simulink model "CryoDet6"  (R2015a)
settings: Solver=ode45  SolverMode=SingleTasking  StartTime=0.0  StopTime=1e-3  MaxStep=Tclk/8  RelTol=1e-3
values from neighbouring files (symbols this model uses):
  Fclk = Fadc/2    (= 185000000)    [setupCryoFPGA.m]    (also in setupCryoNew.m)
  noise = exp(1i*phi)    [setupCryoFPGA.m]    (also in setupCryoNew.m = exp(2i*pi*rand(1, noiseLen)))
  noiseLen = 128    [setupCryoFPGA.m]    (also in setupCryoNew.m)
  noiseSteps = 32    [setupCryoFPGA.m]    (also in setupCryoNew.m)
  notch = tf( [1 a*wNotch/Q wNotch^2], [1 wNotch/Q wNotch^2])    [setupCryoFPGA.m]    (also in setupCryoNew.m)
  notch2 = tf( [1 a*wNotch/Q wNotch^2], [1 wNotch/Q wNotch^2])    [setupCryoFPGA.m]    (also in setupCryoNew.m)
  setupVers = 5    [setupCryoFPGA.m]    (also in setupCryoNew.m = 21)
  Tclk = 1/Fclk    (= 5.40540540541e-09)    [setupCryoFPGA.m]    (also in setupCryoNew.m)
  wTs1 = w1*Ts1    (= 0.0271705310581)    [setupCryoFPGA.m]
undefined symbols (not defined in the file or in its folder): AXI4, Lite, xlipgetpartsetting
libraries: xbsIndex_r4 x516, simulink x1
(part 4 of 6)

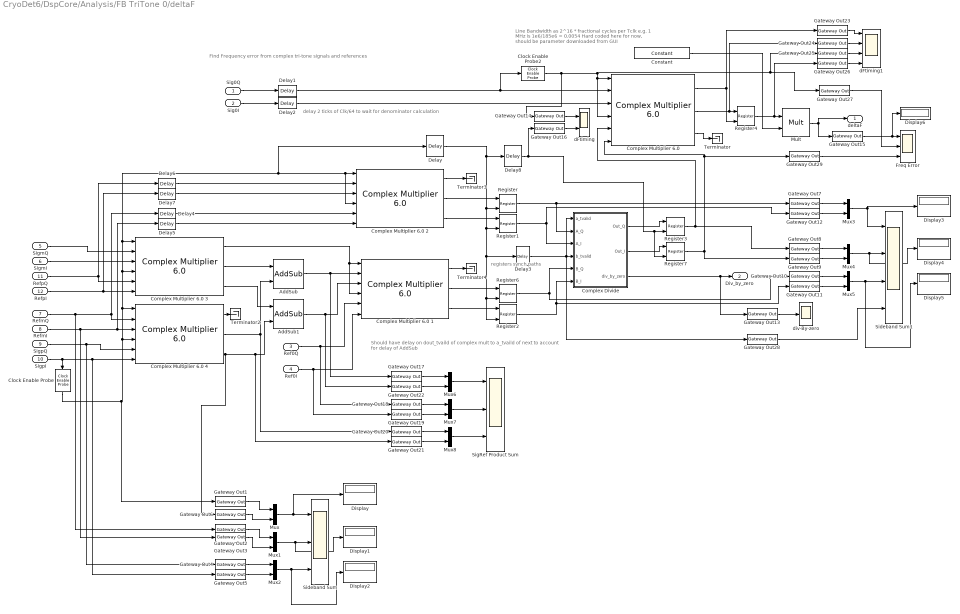
== system CryoDet6/DspCore/Analysis/FB TriTone 0/deltaF ==
  note: Should have delay on dout_tvaild of complex mult to a_tvaild of next
      | to account for delay of AddSub
  note: registers
      | synch
      | paths
  note: delay 2 ticks of Clk/64 to wait for denominator calculation
  note: Line Bandwidth as 2^16 * fractional cycles per Tclk
      | e.g. 1 MHz is 1e6/185e6 = 0.0054
      | Hard coded here for now, should be parameter
      | downloaded from GUI
  note: Find Frequency error from complex tri-tone signals and references
  Sig0Q : Inport
  Sig0I : Inport  Port=2
  Ref0Q : Inport  Port=3
  Ref0I : Inport  Port=4
  SigmQ : Inport  Port=5
  SigmI : Inport  Port=6
  RefmQ : Inport  Port=7
  RefmI : Inport  Port=8
  SigpQ : Inport  Port=9
  SigpI : Inport  Port=10
  RefpQ : Inport  Port=11
  RefpI : Inport  Port=12
  AddSub : xbsIndex_r4/AddSub  mode=Addition  use_carryin=off  use_carryout=off  en=off  latency=3  precision=User Defined  arith_type="Signed  (2's comp)"  n_bits=32  bin_pt=30  quantization=Truncate  overflow=Wrap  use_behavioral_HDL=off  hw_selection=Fabric  pipelined=off  dbl_ovrd=off  block_type=addsub
  AddSub1 : xbsIndex_r4/AddSub  mode=Addition  use_carryin=off  use_carryout=off  en=off  latency=3  precision=User Defined  arith_type="Signed  (2's comp)"  n_bits=32  bin_pt=30  quantization=Truncate  overflow=Wrap  use_behavioral_HDL=off  hw_selection=Fabric  pipelined=off  dbl_ovrd=off  block_type=addsub
  Clock Enable Probe : xbsIndex_r4/Clock Enable Probe  inherit_constraints=on  block_type=ceprobe
      settings: infoedit="Clock enable extractor.  Produces a Boolean output that mirrors the hardware clock enable associated with the input sample rate.<br><br>Hardware notes: in hardware this block costs nothing."
  Clock Enable Probe2 : xbsIndex_r4/Clock Enable Probe  inherit_constraints=on  block_type=ceprobe
      settings: infoedit="Clock enable extractor.  Produces a Boolean output that mirrors the hardware clock enable associated with the input sample rate.<br><br>Hardware notes: in hardware this block costs nothing."
  Complex Divide : Subsystem
  "Complex Multiplier 6.0 " : xbsIndex_r4/Complex Multiplier 6.0   hasatlast=off  hasatuser=off  atuserwidth=1  hasbtlast=off  hasbtuser=off  btuserwidth=1  multtype=Use_Mults  optimizegoal=Resources  flowcontrol=NonBlocking  outputwidth=33  roundmode=Truncate  hasctrltlast=off  hasctrltuser=off  ctrltuserwidth=1  outtlastbehv=Null  latencyconfig=Manual  minimumlatency=37  aclken=off  aresetn=off  trim_axipin_name=on  simulation_type=hybrid_sim  simulation_model=sysgen:cmpy_v6_0  data_path_portlist={ 's_axis_a_tdata_real', 's_axis_a_tdata_imag', 's_axis_b_tdata_real', 's_axis_b_tdata_imag', 's_axis_ctrl_tdata_rounding_bit', 'm_axis_dout_tdata_real', 'm_axis_dout_tdata_imag' }  aportwidth=63  bportwidth=63  ip_name=Complex Multiplier  ip_version=6.0  dsptool_ready=true  ipcore_usecache=true  ipcore_useipmodelcache=true  ipcore_verbose=false  ipcore_latency_parameter='minimumlatency'  wrapper_available=true  port_translation_map={ 'aclken' => 'en', 'aresetn' => 'rst'}  block_type=cmpy_v6_0
  Complex Multiplier 6.0 1 : xbsIndex_r4/Complex Multiplier 6.0   hasatlast=off  hasatuser=off  atuserwidth=1  hasbtlast=off  hasbtuser=off  btuserwidth=1  multtype=Use_Mults  optimizegoal=Resources  flowcontrol=NonBlocking  outputwidth=48  roundmode=Truncate  hasctrltlast=off  hasctrltuser=off  ctrltuserwidth=1  outtlastbehv=Null  latencyconfig=Manual  minimumlatency=37  aclken=off  aresetn=off  trim_axipin_name=on  simulation_type=hybrid_sim  simulation_model=sysgen:cmpy_v6_0  data_path_portlist={ 's_axis_a_tdata_real', 's_axis_a_tdata_imag', 's_axis_b_tdata_real', 's_axis_b_tdata_imag', 's_axis_ctrl_tdata_rounding_bit', 'm_axis_dout_tdata_real', 'm_axis_dout_tdata_imag' }  aportwidth=63  bportwidth=63  ip_name=Complex Multiplier  ip_version=6.0  dsptool_ready=true  ipcore_usecache=true  ipcore_useipmodelcache=true  ipcore_verbose=false  ipcore_latency_parameter='minimumlatency'  wrapper_available=true  port_translation_map={ 'aclken' => 'en', 'aresetn' => 'rst'}  block_type=cmpy_v6_0
  Complex Multiplier 6.0 2 : xbsIndex_r4/Complex Multiplier 6.0   hasatlast=off  hasatuser=off  atuserwidth=1  hasbtlast=off  hasbtuser=off  btuserwidth=1  multtype=Use_Mults  optimizegoal=Resources  flowcontrol=NonBlocking  outputwidth=32  roundmode=Truncate  hasctrltlast=off  hasctrltuser=off  ctrltuserwidth=1  outtlastbehv=Null  latencyconfig=Manual  minimumlatency=37  aclken=off  aresetn=off  trim_axipin_name=on  simulation_type=hybrid_sim  simulation_model=sysgen:cmpy_v6_0  data_path_portlist={ 's_axis_a_tdata_real', 's_axis_a_tdata_imag', 's_axis_b_tdata_real', 's_axis_b_tdata_imag', 's_axis_ctrl_tdata_rounding_bit', 'm_axis_dout_tdata_real', 'm_axis_dout_tdata_imag' }  aportwidth=63  bportwidth=63  ip_name=Complex Multiplier  ip_version=6.0  dsptool_ready=true  ipcore_usecache=true  ipcore_useipmodelcache=true  ipcore_verbose=false  ipcore_latency_parameter='minimumlatency'  wrapper_available=true  port_translation_map={ 'aclken' => 'en', 'aresetn' => 'rst'}  block_type=cmpy_v6_0
  Complex Multiplier 6.0 3 : xbsIndex_r4/Complex Multiplier 6.0   hasatlast=off  hasatuser=off  atuserwidth=1  hasbtlast=off  hasbtuser=off  btuserwidth=1  multtype=Use_Mults  optimizegoal=Resources  flowcontrol=NonBlocking  outputwidth=32  roundmode=Truncate  hasctrltlast=off  hasctrltuser=off  ctrltuserwidth=1  outtlastbehv=Null  latencyconfig=Manual  minimumlatency=37  aclken=off  aresetn=off  trim_axipin_name=on  simulation_type=hybrid_sim  simulation_model=sysgen:cmpy_v6_0  data_path_portlist={ 's_axis_a_tdata_real', 's_axis_a_tdata_imag', 's_axis_b_tdata_real', 's_axis_b_tdata_imag', 's_axis_ctrl_tdata_rounding_bit', 'm_axis_dout_tdata_real', 'm_axis_dout_tdata_imag' }  aportwidth=63  bportwidth=63  ip_name=Complex Multiplier  ip_version=6.0  dsptool_ready=true  ipcore_usecache=true  ipcore_useipmodelcache=true  ipcore_verbose=false  ipcore_latency_parameter='minimumlatency'  wrapper_available=true  port_translation_map={ 'aclken' => 'en', 'aresetn' => 'rst'}  block_type=cmpy_v6_0
  Complex Multiplier 6.0 4 : xbsIndex_r4/Complex Multiplier 6.0   hasatlast=off  hasatuser=off  atuserwidth=1  hasbtlast=off  hasbtuser=off  btuserwidth=1  multtype=Use_Mults  optimizegoal=Resources  flowcontrol=NonBlocking  outputwidth=32  roundmode=Truncate  hasctrltlast=off  hasctrltuser=off  ctrltuserwidth=1  outtlastbehv=Null  latencyconfig=Manual  minimumlatency=37  aclken=off  aresetn=off  trim_axipin_name=on  simulation_type=hybrid_sim  simulation_model=sysgen:cmpy_v6_0  data_path_portlist={ 's_axis_a_tdata_real', 's_axis_a_tdata_imag', 's_axis_b_tdata_real', 's_axis_b_tdata_imag', 's_axis_ctrl_tdata_rounding_bit', 'm_axis_dout_tdata_real', 'm_axis_dout_tdata_imag' }  aportwidth=63  bportwidth=63  ip_name=Complex Multiplier  ip_version=6.0  dsptool_ready=true  ipcore_usecache=true  ipcore_useipmodelcache=true  ipcore_verbose=false  ipcore_latency_parameter='minimumlatency'  wrapper_available=true  port_translation_map={ 'aclken' => 'en', 'aresetn' => 'rst'}  block_type=cmpy_v6_0
  Constant : xbsIndex_r4/Constant  const=1e6/Fclk  gui_display_data_type=Fixed-point  arith_type=Unsigned  n_bits=16  bin_pt=16  preci_type=Single  exp_width=8  frac_width=24  explicit_period=off  period=1  equ=P=C  opselect=C  inp2=PCIN>>17  opr=+  inp1=P  carry=CIN  dbl_ovrd=off  block_type=constant
  Delay : xbsIndex_r4/Delay  rst=off  infoeditControl=Selection of Reset will increase slice count due to use of real FFs and instead of SRLs  en=off  latency=80  reg_retiming=off  dbl_ovrd=off  block_type=delay
  Delay1 : xbsIndex_r4/Delay  rst=off  infoeditControl=Selection of Reset will increase slice count due to use of real FFs and instead of SRLs  en=off  latency=3  reg_retiming=off  dbl_ovrd=off  block_type=delay
  Delay2 : xbsIndex_r4/Delay  rst=off  infoeditControl=Selection of Reset will increase slice count due to use of real FFs and instead of SRLs  en=off  latency=3  reg_retiming=off  dbl_ovrd=off  block_type=delay
  Delay3 : xbsIndex_r4/Delay  rst=off  infoeditControl=Selection of Reset will increase slice count due to use of real FFs and instead of SRLs  en=off  latency=2  reg_retiming=off  dbl_ovrd=off  block_type=delay
  Delay{4..7} (4 alike) : xbsIndex_r4/Delay  rst=off  infoeditControl=Selection of Reset will increase slice count due to use of real FFs and instead of SRLs  en=off  latency=2  reg_retiming=on  dbl_ovrd=off  block_type=delay
  Delay8 : xbsIndex_r4/Delay  rst=off  infoeditControl=Selection of Reset will increase slice count due to use of real FFs and instead of SRLs  en=off  latency=104  reg_retiming=off  dbl_ovrd=off  block_type=delay
  Display{,1..6} (7 alike) : Display
  Freq Error : Scope  NumInputPorts=3
      settings: TimeRange=6.023783783783785e-05  YMin=0.0075~0~-3.725  YMax=0.01025~1~-3.175  SaveName=ScopeData12
  Gateway Out{1..29} (29 alike) : xbsIndex_r4/Gateway Out  inherit_from_input=off  hdl_port=off  rows=1  columns=1  UseAsDAC=off  DACChannel='1'  interface=None  automatic_assignment=on  address_offset=hex2dec('00')  intf_name=''  intf_description=''  timing_constraint=None  locs_specified=off  LOCs={}  io_standard={}  block_type=gatewayout
  Mult : xbsIndex_r4/Mult  precision=User Defined  arith_type="Signed  (2's comp)"  n_bits=24  bin_pt=22  quantization=Truncate  overflow=Saturate  en=off  latency=3  use_behavioral_HDL=off  opt=Speed  use_embedded=on  optimum_pipeline=off  pipeline=on  dbl_ovrd=off  use_rpm=on  placement_style=Triangular  block_type=mult
  Mux{,1..8} (9 alike) : Mux  Inputs=2
  Register{,1..4,6..7} (7 alike) : xbsIndex_r4/Register  init=0  rst=off  en=on  dbl_ovrd=off  block_type=register
  Sideband Sum : Scope  NumInputPorts=3
      settings: YMin=-0.1~-0.045~-0.0015  YMax=1~0.02~0.0045  SaveName=ScopeData2
  Sideband Sum1 : Scope  NumInputPorts=4
      settings: YMin=-0.02~-4~-0.02~0  YMax=0.14~4~0.02~1  SaveName=ScopeData4
  SigRef Product Sum : Scope  NumInputPorts=3
      settings: YMin=-0.009~-0.005~-0.004  YMax=0.007~0.075~0.00075  SaveName=ScopeData9
  Terminator{,2..4} (4 alike) : Terminator
  dFtiming : Scope  NumInputPorts=2
      settings: TimeRange=2e-05  YMin=-0.00225~0  YMax=0.0015~1  SaveName=ScopeData14
  dFtiming1 : Scope  NumInputPorts=4
      settings: YMin=0~-1~0~-1  YMax=1~2.5~1~2.5  SaveName=ScopeData15
  div-By-zero : Scope
      settings: YMin=-0.15  YMax=0.9  SaveName=ScopeData5
  deltaF : Outport
  Div_by_zero : Outport  Port=2
  wires:
  "Complex Multiplier 6.0 "/2 -> Gateway Out24/1, Register4/1
  Mult/1 -> deltaF/1, Gateway Out15/1
  Constant/1 -> Mult/2
  Complex Divide/1(Out_Q) -> Register3/1
  Complex Divide/2(Out_I) -> Register7/1
  Sig0Q/1 -> Delay1/1
  Sig0I/1 -> Delay2/1
  "Complex Multiplier 6.0 "/3 -> Terminator/1
  "Complex Multiplier 6.0 "/1 -> Register4/2, Gateway Out23/1
  Complex Multiplier 6.0 3/2 -> AddSub/1
  Complex Multiplier 6.0 4/2 -> Gateway Out20/1, AddSub/2
  Complex Multiplier 6.0 3/3 -> AddSub1/1
  Complex Multiplier 6.0 4/3 -> Gateway Out6/1, Gateway Out21/1, AddSub1/2
  AddSub/1 -> Gateway Out17/1, Complex Multiplier 6.0 1/2
  AddSub1/1 -> Gateway Out22/1, Complex Multiplier 6.0 1/3
  Ref0Q/1 -> Gateway Out18/1, Complex Multiplier 6.0 1/5
  Complex Multiplier 6.0 1/2 -> Register6/1
  Complex Multiplier 6.0 1/3 -> Register2/1
  Complex Multiplier 6.0 2/2 -> Register/1
  Complex Multiplier 6.0 2/3 -> Register1/1
  SigmI/1 -> Complex Multiplier 6.0 3/3
  SigmQ/1 -> Complex Multiplier 6.0 3/2
  SigpI/1 -> Gateway Out5/1, Complex Multiplier 6.0 4/6, Clock Enable Probe/1
  SigpQ/1 -> Gateway Out4/1, Complex Multiplier 6.0 4/5
  RefmQ/1 -> Gateway Out2/1, Complex Multiplier 6.0 4/2, Delay4/1
  RefmI/1 -> Gateway Out3/1, Complex Multiplier 6.0 4/3, Delay5/1
  RefpI/1 -> Complex Multiplier 6.0 3/6, Delay7/1
  RefpQ/1 -> Delay6/1, Complex Multiplier 6.0 3/5
  Clock Enable Probe/1 -> Gateway Out1/1, Complex Multiplier 6.0 4/4, Complex Multiplier 6.0 4/1, Complex Multiplier 6.0 3/4, Delay/1, Complex Multiplier 6.0 2/4, Complex Multiplier 6.0 2/1, Complex Multiplier 6.0 3/1
  Complex Multiplier 6.0 3/1 -> Complex Multiplier 6.0 1/4, Complex Multiplier 6.0 1/1
  Complex Multiplier 6.0 4/1 -> Terminator2/1
  Clock Enable Probe2/1 -> Gateway Out14/1, "Complex Multiplier 6.0 "/4, "Complex Multiplier 6.0 "/1, Gateway Out25/1, Gateway Out27/1
  Gateway Out2/1 -> Mux1/1
  Gateway Out3/1 -> Mux1/2
  Gateway Out4/1 -> Mux2/1
  Gateway Out5/1 -> Mux2/2
  Mux/1 -> Display/1, Sideband Sum/1
  Mux1/1 -> Display1/1, Sideband Sum/2
  Mux2/1 -> Display2/1, Sideband Sum/3
  Gateway Out1/1 -> Mux/1
  Gateway Out6/1 -> Mux/2
  Ref0I/1 -> Gateway Out19/1, Complex Multiplier 6.0 1/6
  Gateway Out8/1 -> Mux4/1
  Gateway Out9/1 -> Mux4/2
  Gateway Out10/1 -> Mux5/1
  Gateway Out11/1 -> Mux5/2
  Mux3/1 -> Sideband Sum1/1, Display3/1
  Mux4/1 -> Display4/1, Sideband Sum1/2
  Mux5/1 -> Display5/1, Sideband Sum1/3
  Gateway Out7/1 -> Mux3/1
  Gateway Out12/1 -> Mux3/2
  Complex Divide/3(div_by_zero) -> Div_by_zero/1, Gateway Out13/1
  Complex Multiplier 6.0 2/1 -> Terminator3/1
  Complex Multiplier 6.0 1/1 -> Terminator4/1
  Gateway Out13/1 -> div-By-zero/1
  Delay/1 -> Delay8/1, Register6/2, Register2/2, Delay3/1, Register1/2, Register/2
  Delay1/1 -> Clock Enable Probe2/1, "Complex Multiplier 6.0 "/2
  Delay2/1 -> "Complex Multiplier 6.0 "/3
  Delay5/1 -> Complex Multiplier 6.0 2/6
  Delay4/1 -> Complex Multiplier 6.0 2/5
  Delay7/1 -> Complex Multiplier 6.0 2/3
  Delay6/1 -> Complex Multiplier 6.0 2/2
  Delay3/1 -> Complex Divide/1(a_tvalid), Gateway Out28/1, Complex Divide/4(b_tvalid)
  Gateway Out15/1 -> Display6/1, Freq Error/1
  Register3/1 -> Gateway Out8/1, "Complex Multiplier 6.0 "/5
  Register7/1 -> Gateway Out29/1, "Complex Multiplier 6.0 "/6, Gateway Out9/1
  Delay8/1 -> Gateway Out16/1, Register7/2, Register3/2
  Gateway Out14/1 -> dFtiming/1
  Gateway Out16/1 -> dFtiming/2
  Gateway Out18/1 -> Mux7/1
  Gateway Out19/1 -> Mux7/2
  Gateway Out20/1 -> Mux8/1
  Gateway Out21/1 -> Mux8/2
  Mux6/1 -> SigRef Product Sum/1
  Mux7/1 -> SigRef Product Sum/2
  Mux8/1 -> SigRef Product Sum/3
  Gateway Out17/1 -> Mux6/1
  Gateway Out22/1 -> Mux6/2
  Gateway Out23/1 -> dFtiming1/1
  Gateway Out24/1 -> dFtiming1/2
  Gateway Out25/1 -> dFtiming1/3
  Register4/1 -> Gateway Out26/1, Mult/1
  Gateway Out26/1 -> dFtiming1/4
  Register/1 -> Complex Divide/2(A_Q), Gateway Out7/1
  Register1/1 -> Complex Divide/3(A_I), Gateway Out12/1
  Register6/1 -> Gateway Out10/1, Complex Divide/5(B_Q)
  Register2/1 -> Gateway Out11/1, Complex Divide/6(B_I)
  Gateway Out27/1 -> Freq Error/2
  Gateway Out28/1 -> Sideband Sum1/4
  Gateway Out29/1 -> Freq Error/3

== system CryoDet6/DspCore/Analysis/FB TriTone 0/toneGen ==
  Freq : Inport
  Constant : xbsIndex_r4/Constant  const=1.0  gui_display_data_type=Boolean  arith_type=Boolean  n_bits=16  bin_pt=14  preci_type=Single  exp_width=8  frac_width=24  explicit_period=off  period=1  equ=P=C  opselect=C  inp2=PCIN>>17  opr=+  inp1=P  carry=CIN  dbl_ovrd=off  block_type=constant
  "DDS Compiler 6.0 " : xbsIndex_r4/DDS Compiler 6.0   partspresent=Phase_Generator_and_SIN_COS_LUT  dds_clock_rate=Fclk/1e6  channels=1  mode_of_operation=Standard  modulus=9  parameter_entry=Hardware_Parameters  spurious_free_dynamic_range=45  frequency_resolution=0.4  noise_shaping=None  phase_width=16  output_width=16  output_selection=Sine_and_Cosine  negative_sine=off  negative_cosine=off  amplitude_mode=Unit_Circle  memory_type=Auto  optimization_goal=Speed  dsp48_use=Maximal  resync=off  latency_configuration=Configurable  latency=15  has_phase_out=off  has_aclken=off  has_aresetn=off  explicit_period=on  period=Tclk  data_has_tlast=Not_Required  has_tready=off  s_phase_has_tuser=Not_Required  m_data_has_tuser=Not_Required  m_phase_has_tuser=Not_Required  s_phase_tuser_width=1  output_form=Twos_Complement  s_config_sync_mode=On_Vector  phase_increment=Programmable  output_frequency1=0  output_frequency2=0  output_frequency3=0  output_frequency4=0  output_frequency5=0  output_frequency6=0  output_frequency7=0  output_frequency8=0  output_frequency9=0  output_frequency10=0  output_frequency11=0  output_frequency12=0  output_frequency13=0  output_frequency14=0  output_frequency15=0  output_frequency16=0  pinc1='0'  pinc2='0'  pinc3='0'  pinc4='0'  pinc5='0'  pinc6='0'  pinc7='0'  pinc8='0'  pinc9='0'  pinc10='0'  pinc11='0'  pinc12='0'  pinc13='0'  pinc14='0'  pinc15='0'  pinc16='0'  phase_offset=None  phase_offset_angles1=0  phase_offset_angles2=0  phase_offset_angles3=0  phase_offset_angles4=0  phase_offset_angles5=0  phase_offset_angles6=0  phase_offset_angles7=0  phase_offset_angles8=0  phase_offset_angles9=0  phase_offset_angles10=0  phase_offset_angles11=0  phase_offset_angles12=0  phase_offset_angles13=0  phase_offset_angles14=0  phase_offset_angles15=0  phase_offset_angles16=0  poff1='0'  poff2='0'  poff3='0'  poff4='0'  poff5='0'  poff6='0'  poff7='0'  poff8='0'  poff9='0'  poff10='0'  poff11='0'  poff12='0'  poff13='0'  poff14='0'  poff15='0'  poff16='0'  trim_axipin_name=on  simulation_type=hybrid_sim  simulation_model=sysgen:xddsv6_0_cmodel  data_path_portlist={ 's_axis_config_tdata_poff', 's_axis_config_tdata_chan0_poff', 's_axis_config_tdata_pinc', 's_axis_config_tdata_chan0_pinc', 's_axis_phase_tdata_resync', 's_axis_phase_tdata_chan0_resync', 's_axis_phase_tdata_poff', 's_axis_phase_tdata_chan0_poff', 's_axis_phase_tdata_pinc', 's_axis_phase_tdata_chan0_pinc', 's_axis_phase_tdata_phase_in', 'm_axis_data_tdata_sine', 'm_axis_data_tdata_chan0_sine', 'm_axis_data_tdata_cosine', 'm_axis_data_tdata_chan0_cosine', 'm_axis_phase_tdata_phase_out', 'm_axis_phase_tdata_chan0_phase_out'}  por_mode=false  gui_behaviour=Sysgen  ip_name=DDS Compiler  ip_version=6.0  dsptool_ready=true  wrapper_available=true  port_translation_map={ 'aclken' => 'en', 'aresetn' => 'rst' }  ipcore_usecache=true  ipcore_useipmodelcache=true  ipcore_xco_need_fpga_part=true  ipcore_fpga_part=xlipgetpartsetting(gcb, {'kintex7', 'xc7k325t', '-3', 'fbg676'})  ipcore_verbose=false  block_type=dds_compiler_v6_0
  Display : Display
  Display1 : Display
  Gateway Out : xbsIndex_r4/Gateway Out  inherit_from_input=off  hdl_port=off  rows=1  columns=1  UseAsDAC=off  DACChannel='1'  interface=None  automatic_assignment=on  address_offset=hex2dec('00')  intf_name=''  intf_description=''  timing_constraint=None  locs_specified=off  LOCs={}  io_standard={}  block_type=gatewayout
  Gateway Out1 : xbsIndex_r4/Gateway Out  inherit_from_input=off  hdl_port=off  rows=1  columns=1  UseAsDAC=off  DACChannel='1'  interface=None  automatic_assignment=on  address_offset=hex2dec('00')  intf_name=''  intf_description=''  timing_constraint=None  locs_specified=off  LOCs={}  io_standard={}  block_type=gatewayout
  Gateway Out2 : xbsIndex_r4/Gateway Out  inherit_from_input=off  hdl_port=off  rows=1  columns=1  UseAsDAC=off  DACChannel='1'  interface=None  automatic_assignment=on  address_offset=hex2dec('00')  intf_name=''  intf_description=''  timing_constraint=None  locs_specified=off  LOCs={}  io_standard={}  block_type=gatewayout
  Mult : xbsIndex_r4/Mult  precision=User Defined  arith_type="Signed  (2's comp)"  n_bits=16  bin_pt=15  quantization=Truncate  overflow=Wrap  en=off  latency=3  use_behavioral_HDL=off  opt=Speed  use_embedded=on  optimum_pipeline=off  pipeline=on  dbl_ovrd=off  use_rpm=on  placement_style=Triangular  block_type=mult
  Mult1 : xbsIndex_r4/Mult  precision=User Defined  arith_type="Signed  (2's comp)"  n_bits=16  bin_pt=15  quantization=Truncate  overflow=Wrap  en=off  latency=3  use_behavioral_HDL=off  opt=Speed  use_embedded=on  optimum_pipeline=off  pipeline=on  dbl_ovrd=off  use_rpm=on  placement_style=Triangular  block_type=mult
  Mux : Mux  Inputs=2
  Reinterpret : xbsIndex_r4/Reinterpret  force_arith_type=on  arith_type=Unsigned  force_bin_pt=off  bin_pt=0  block_type=reinterpret
  Terminator : Terminator
  IFI : Outport
  IFQ : Outport  Port=2
  wires:
  Freq/1 -> Gateway Out/1, Reinterpret/1
  Constant/1 -> "DDS Compiler 6.0 "/1
  "DDS Compiler 6.0 "/2 -> Mult1/1
  "DDS Compiler 6.0 "/3 -> Mult/2
  [Ampl0] -> Gateway Out1/1, Mult1/2, Mult/1
  Mult/1 -> IFI/1
  Mult1/1 -> IFQ/1
  "DDS Compiler 6.0 "/1 -> Terminator/1
  Gateway Out1/1 -> Display1/1
  Reinterpret/1 -> Gateway Out2/1, "DDS Compiler 6.0 "/2
  Gateway Out/1 -> Mux/1
  Gateway Out2/1 -> Mux/2
  Mux/1 -> Display/1

== system CryoDet6/DspCore/Analysis/sidebands/Phase Modulator ==
  Iin : Inport
  Qin : Inport  Port=2
  Ipm : Inport  Port=3
  Qpm : Inport  Port=4
  AddSub : xbsIndex_r4/AddSub  mode=Subtraction  use_carryin=off  use_carryout=off  en=off  latency=1  precision=User Defined  arith_type="Signed  (2's comp)"  n_bits=16  bin_pt=15  quantization=Truncate  overflow=Wrap  use_behavioral_HDL=off  hw_selection=Fabric  pipelined=off  dbl_ovrd=off  block_type=addsub
  AddSub1 : xbsIndex_r4/AddSub  mode=Addition  use_carryin=off  use_carryout=off  en=off  latency=1  precision=User Defined  arith_type="Signed  (2's comp)"  n_bits=16  bin_pt=15  quantization=Truncate  overflow=Wrap  use_behavioral_HDL=off  hw_selection=Fabric  pipelined=off  dbl_ovrd=off  block_type=addsub
  Mult{1..4} (4 alike) : xbsIndex_r4/Mult  precision=User Defined  arith_type="Signed  (2's comp)"  n_bits=16  bin_pt=15  quantization=Truncate  overflow=Wrap  en=off  latency=3  use_behavioral_HDL=off  opt=Speed  use_embedded=on  optimum_pipeline=off  pipeline=on  dbl_ovrd=off  use_rpm=on  placement_style=Triangular  block_type=mult
  Iout : Outport
  Qout : Outport  Port=2
  wires:
  Iin/1 -> Mult4/1, Mult2/1
  Qin/1 -> Mult1/1, Mult3/1
  Ipm/1 -> Mult2/2, Mult1/2
  Qpm/1 -> Mult3/2, Mult4/2
  Mult2/1 -> AddSub/1
  Mult3/1 -> AddSub/2
  Mult1/1 -> AddSub1/1
  Mult4/1 -> AddSub1/2
  AddSub/1 -> Iout/1
  AddSub1/1 -> Qout/1

== system CryoDet6/DspCore/Analysis/FB TriTone 0/TriTone Downconvert/CIC Filter ==
  note: The CIC filter is constructed out of differentiators and integrators and
      | a sample rate change. This block provides a full precision result and is
      | dynamically built given the parameters entered in the dialog box. The
      | dynamic rebuilding script can switch which side the integrators and
      | differentiators are on and also change between an up and down sampler
      | depending on whether an Interpolator or decimator is selected respectively.
      | The number of stages selected control how many integrators and
      | differentiators are used.
  note: The Interpoiation by 48, 4 stage CIC filter occupies 116 slices.
      | The maximum clock frequency is approximately
      | 308.55 MHz in a Xilinx xc2vp2-7 part (Device speed data version:
      | PRODUCTION 1.121 2005-11-04, ISE 8.1.01i I.25 software, VHDL
      | synthesized with XST).
  In1 : Inport
  Differentiator1 : Subsystem  mask(Differentiator Stage){m=m, output_bitwidth=ceil(stages*log2(rate_change*m) + input_bitwidth), output_binpt=input_binpt}
      mask prompts: m "Differential Delay"; output_bitwidth "Output Bit Width"; output_binpt "Output Binary Point"
      mask help: Multi-Channel Differentiator
      mask init:
      | set_param(gcb, 'LinkStatus', 'none');
  Differentiator2 : Subsystem  mask(Differentiator Stage){m=m, output_bitwidth=ceil(stages*log2(rate_change*m) + input_bitwidth), output_binpt=input_binpt}
      mask prompts: m "Differential Delay"; output_bitwidth "Output Bit Width"; output_binpt "Output Binary Point"
      mask help: Multi-Channel Differentiator
      mask init:
      | set_param(gcb, 'LinkStatus', 'none');
  Differentiator3 : Subsystem  mask(Differentiator Stage){m=m, output_bitwidth=ceil(stages*log2(rate_change*m) + input_bitwidth), output_binpt=input_binpt}
      mask prompts: m "Differential Delay"; output_bitwidth "Output Bit Width"; output_binpt "Output Binary Point"
      mask help: Multi-Channel Differentiator
      mask init:
      | set_param(gcb, 'LinkStatus', 'none');
  Down Sample : xbsIndex_r4/Down Sample  sample_ratio=rate_change  sample_phase=First Value of Frame  en=off  rst=off  latency=1  dbl_ovrd=off  block_type=dsamp
      settings: block_version=9.2.00
  Integrator1 : Subsystem  mask(Integrator Stage){output_bitwidth=ceil(stages*log2(rate_change*m) + input_bitwidth)}
      mask prompts: output_bitwidth "Output Bit Width"
      mask help: Multi Channel Integrator
      mask init:
      | set_param(gcb, 'LinkStatus', 'none');
      settings: CopyFcn=set_param(gcb, 'LinkStatus', 'none');
  Integrator2 : Subsystem  mask(Integrator Stage){output_bitwidth=ceil(stages*log2(rate_change*m) + input_bitwidth)}
      mask prompts: output_bitwidth "Output Bit Width"
      mask help: Multi Channel Integrator
      mask init:
      | set_param(gcb, 'LinkStatus', 'none');
      settings: CopyFcn=set_param(gcb, 'LinkStatus', 'none');
  Integrator3 : Subsystem  mask(Integrator Stage){output_bitwidth=ceil(stages*log2(rate_change*m) + input_bitwidth)}
      mask prompts: output_bitwidth "Output Bit Width"
      mask help: Multi Channel Integrator
      mask init:
      | set_param(gcb, 'LinkStatus', 'none');
      settings: CopyFcn=set_param(gcb, 'LinkStatus', 'none');
  Out1 : Outport
  wires:
  In1/1 -> Integrator1/1(In1)
  Down Sample/1 -> Differentiator1/1(In1)
  Integrator1/1(Out1) -> Integrator2/1(In1)
  Differentiator1/1(Out1) -> Differentiator2/1(In1)
  Integrator2/1(Out1) -> Integrator3/1(In1)
  Differentiator2/1(Out1) -> Differentiator3/1(In1)
  Integrator3/1(Out1) -> Down Sample/1
  Differentiator3/1(Out1) -> Out1/1

== system CryoDet6/DspCore/Analysis/FB TriTone 0/TriTone Downconvert/CIC Filter1 ==
  note: The CIC filter is constructed out of differentiators and integrators and
      | a sample rate change. This block provides a full precision result and is
      | dynamically built given the parameters entered in the dialog box. The
      | dynamic rebuilding script can switch which side the integrators and
      | differentiators are on and also change between an up and down sampler
      | depending on whether an Interpolator or decimator is selected respectively.
      | The number of stages selected control how many integrators and
      | differentiators are used.
  note: The Interpoiation by 48, 4 stage CIC filter occupies 116 slices.
      | The maximum clock frequency is approximately
      | 308.55 MHz in a Xilinx xc2vp2-7 part (Device speed data version:
      | PRODUCTION 1.121 2005-11-04, ISE 8.1.01i I.25 software, VHDL
      | synthesized with XST).
  In1 : Inport
  Differentiator1 : Subsystem  mask(Differentiator Stage){m=m, output_bitwidth=ceil(stages*log2(rate_change*m) + input_bitwidth), output_binpt=input_binpt}
      mask prompts: m "Differential Delay"; output_bitwidth "Output Bit Width"; output_binpt "Output Binary Point"
      mask help: Multi-Channel Differentiator
      mask init:
      | set_param(gcb, 'LinkStatus', 'none');
  Differentiator2 : Subsystem  mask(Differentiator Stage){m=m, output_bitwidth=ceil(stages*log2(rate_change*m) + input_bitwidth), output_binpt=input_binpt}
      mask prompts: m "Differential Delay"; output_bitwidth "Output Bit Width"; output_binpt "Output Binary Point"
      mask help: Multi-Channel Differentiator
      mask init:
      | set_param(gcb, 'LinkStatus', 'none');
  Differentiator3 : Subsystem  mask(Differentiator Stage){m=m, output_bitwidth=ceil(stages*log2(rate_change*m) + input_bitwidth), output_binpt=input_binpt}
      mask prompts: m "Differential Delay"; output_bitwidth "Output Bit Width"; output_binpt "Output Binary Point"
      mask help: Multi-Channel Differentiator
      mask init:
      | set_param(gcb, 'LinkStatus', 'none');
  Down Sample : xbsIndex_r4/Down Sample  sample_ratio=rate_change  sample_phase=First Value of Frame  en=off  rst=off  latency=1  dbl_ovrd=off  block_type=dsamp
      settings: block_version=9.2.00
  Integrator1 : Subsystem  mask(Integrator Stage){output_bitwidth=ceil(stages*log2(rate_change*m) + input_bitwidth)}
      mask prompts: output_bitwidth "Output Bit Width"
      mask help: Multi Channel Integrator
      mask init:
      | set_param(gcb, 'LinkStatus', 'none');
      settings: CopyFcn=set_param(gcb, 'LinkStatus', 'none');
  Integrator2 : Subsystem  mask(Integrator Stage){output_bitwidth=ceil(stages*log2(rate_change*m) + input_bitwidth)}
      mask prompts: output_bitwidth "Output Bit Width"
      mask help: Multi Channel Integrator
      mask init:
      | set_param(gcb, 'LinkStatus', 'none');
      settings: CopyFcn=set_param(gcb, 'LinkStatus', 'none');
  Integrator3 : Subsystem  mask(Integrator Stage){output_bitwidth=ceil(stages*log2(rate_change*m) + input_bitwidth)}
      mask prompts: output_bitwidth "Output Bit Width"
      mask help: Multi Channel Integrator
      mask init:
      | set_param(gcb, 'LinkStatus', 'none');
      settings: CopyFcn=set_param(gcb, 'LinkStatus', 'none');
  Out1 : Outport
  wires:
  In1/1 -> Integrator1/1(In1)
  Down Sample/1 -> Differentiator1/1(In1)
  Integrator1/1(Out1) -> Integrator2/1(In1)
  Differentiator1/1(Out1) -> Differentiator2/1(In1)
  Integrator2/1(Out1) -> Integrator3/1(In1)
  Differentiator2/1(Out1) -> Differentiator3/1(In1)
  Integrator3/1(Out1) -> Down Sample/1
  Differentiator3/1(Out1) -> Out1/1

== system CryoDet6/DspCore/Analysis/FB TriTone 0/TriTone Downconvert/CIC Filter2 ==
  note: The CIC filter is constructed out of differentiators and integrators and
      | a sample rate change. This block provides a full precision result and is
      | dynamically built given the parameters entered in the dialog box. The
      | dynamic rebuilding script can switch which side the integrators and
      | differentiators are on and also change between an up and down sampler
      | depending on whether an Interpolator or decimator is selected respectively.
      | The number of stages selected control how many integrators and
      | differentiators are used.
  note: The Interpoiation by 48, 4 stage CIC filter occupies 116 slices.
      | The maximum clock frequency is approximately
      | 308.55 MHz in a Xilinx xc2vp2-7 part (Device speed data version:
      | PRODUCTION 1.121 2005-11-04, ISE 8.1.01i I.25 software, VHDL
      | synthesized with XST).
  In1 : Inport
  Differentiator1 : Subsystem  mask(Differentiator Stage){m=m, output_bitwidth=ceil(stages*log2(rate_change*m) + input_bitwidth), output_binpt=input_binpt}
      mask prompts: m "Differential Delay"; output_bitwidth "Output Bit Width"; output_binpt "Output Binary Point"
      mask help: Multi-Channel Differentiator
      mask init:
      | set_param(gcb, 'LinkStatus', 'none');
  Differentiator2 : Subsystem  mask(Differentiator Stage){m=m, output_bitwidth=ceil(stages*log2(rate_change*m) + input_bitwidth), output_binpt=input_binpt}
      mask prompts: m "Differential Delay"; output_bitwidth "Output Bit Width"; output_binpt "Output Binary Point"
      mask help: Multi-Channel Differentiator
      mask init:
      | set_param(gcb, 'LinkStatus', 'none');
  Differentiator3 : Subsystem  mask(Differentiator Stage){m=m, output_bitwidth=ceil(stages*log2(rate_change*m) + input_bitwidth), output_binpt=input_binpt}
      mask prompts: m "Differential Delay"; output_bitwidth "Output Bit Width"; output_binpt "Output Binary Point"
      mask help: Multi-Channel Differentiator
      mask init:
      | set_param(gcb, 'LinkStatus', 'none');
  Down Sample : xbsIndex_r4/Down Sample  sample_ratio=rate_change  sample_phase=First Value of Frame  en=off  rst=off  latency=1  dbl_ovrd=off  block_type=dsamp
      settings: block_version=9.2.00
  Integrator1 : Subsystem  mask(Integrator Stage){output_bitwidth=ceil(stages*log2(rate_change*m) + input_bitwidth)}
      mask prompts: output_bitwidth "Output Bit Width"
      mask help: Multi Channel Integrator
      mask init:
      | set_param(gcb, 'LinkStatus', 'none');
      settings: CopyFcn=set_param(gcb, 'LinkStatus', 'none');
  Integrator2 : Subsystem  mask(Integrator Stage){output_bitwidth=ceil(stages*log2(rate_change*m) + input_bitwidth)}
      mask prompts: output_bitwidth "Output Bit Width"
      mask help: Multi Channel Integrator
      mask init:
      | set_param(gcb, 'LinkStatus', 'none');
      settings: CopyFcn=set_param(gcb, 'LinkStatus', 'none');
  Integrator3 : Subsystem  mask(Integrator Stage){output_bitwidth=ceil(stages*log2(rate_change*m) + input_bitwidth)}
      mask prompts: output_bitwidth "Output Bit Width"
      mask help: Multi Channel Integrator
      mask init:
      | set_param(gcb, 'LinkStatus', 'none');
      settings: CopyFcn=set_param(gcb, 'LinkStatus', 'none');
  Out1 : Outport
  wires:
  In1/1 -> Integrator1/1(In1)
  Down Sample/1 -> Differentiator1/1(In1)
  Integrator1/1(Out1) -> Integrator2/1(In1)
  Differentiator1/1(Out1) -> Differentiator2/1(In1)
  Integrator2/1(Out1) -> Integrator3/1(In1)
  Differentiator2/1(Out1) -> Differentiator3/1(In1)
  Integrator3/1(Out1) -> Down Sample/1
  Differentiator3/1(Out1) -> Out1/1

== system CryoDet6/DspCore/Analysis/FB TriTone 0/TriTone Downconvert/CIC Filter3 ==
  note: The CIC filter is constructed out of differentiators and integrators and
      | a sample rate change. This block provides a full precision result and is
      | dynamically built given the parameters entered in the dialog box. The
      | dynamic rebuilding script can switch which side the integrators and
      | differentiators are on and also change between an up and down sampler
      | depending on whether an Interpolator or decimator is selected respectively.
      | The number of stages selected control how many integrators and
      | differentiators are used.
  note: The Interpoiation by 48, 4 stage CIC filter occupies 116 slices.
      | The maximum clock frequency is approximately
      | 308.55 MHz in a Xilinx xc2vp2-7 part (Device speed data version:
      | PRODUCTION 1.121 2005-11-04, ISE 8.1.01i I.25 software, VHDL
      | synthesized with XST).
  In1 : Inport
  Differentiator1 : Subsystem  mask(Differentiator Stage){m=m, output_bitwidth=ceil(stages*log2(rate_change*m) + input_bitwidth), output_binpt=input_binpt}
      mask prompts: m "Differential Delay"; output_bitwidth "Output Bit Width"; output_binpt "Output Binary Point"
      mask help: Multi-Channel Differentiator
      mask init:
      | set_param(gcb, 'LinkStatus', 'none');
  Differentiator2 : Subsystem  mask(Differentiator Stage){m=m, output_bitwidth=ceil(stages*log2(rate_change*m) + input_bitwidth), output_binpt=input_binpt}
      mask prompts: m "Differential Delay"; output_bitwidth "Output Bit Width"; output_binpt "Output Binary Point"
      mask help: Multi-Channel Differentiator
      mask init:
      | set_param(gcb, 'LinkStatus', 'none');
  Differentiator3 : Subsystem  mask(Differentiator Stage){m=m, output_bitwidth=ceil(stages*log2(rate_change*m) + input_bitwidth), output_binpt=input_binpt}
      mask prompts: m "Differential Delay"; output_bitwidth "Output Bit Width"; output_binpt "Output Binary Point"
      mask help: Multi-Channel Differentiator
      mask init:
      | set_param(gcb, 'LinkStatus', 'none');
  Down Sample : xbsIndex_r4/Down Sample  sample_ratio=rate_change  sample_phase=First Value of Frame  en=off  rst=off  latency=1  dbl_ovrd=off  block_type=dsamp
      settings: block_version=9.2.00
  Integrator1 : Subsystem  mask(Integrator Stage){output_bitwidth=ceil(stages*log2(rate_change*m) + input_bitwidth)}
      mask prompts: output_bitwidth "Output Bit Width"
      mask help: Multi Channel Integrator
      mask init:
      | set_param(gcb, 'LinkStatus', 'none');
      settings: CopyFcn=set_param(gcb, 'LinkStatus', 'none');
  Integrator2 : Subsystem  mask(Integrator Stage){output_bitwidth=ceil(stages*log2(rate_change*m) + input_bitwidth)}
      mask prompts: output_bitwidth "Output Bit Width"
      mask help: Multi Channel Integrator
      mask init:
      | set_param(gcb, 'LinkStatus', 'none');
      settings: CopyFcn=set_param(gcb, 'LinkStatus', 'none');
  Integrator3 : Subsystem  mask(Integrator Stage){output_bitwidth=ceil(stages*log2(rate_change*m) + input_bitwidth)}
      mask prompts: output_bitwidth "Output Bit Width"
      mask help: Multi Channel Integrator
      mask init:
      | set_param(gcb, 'LinkStatus', 'none');
      settings: CopyFcn=set_param(gcb, 'LinkStatus', 'none');
  Out1 : Outport
  wires:
  In1/1 -> Integrator1/1(In1)
  Down Sample/1 -> Differentiator1/1(In1)
  Integrator1/1(Out1) -> Integrator2/1(In1)
  Differentiator1/1(Out1) -> Differentiator2/1(In1)
  Integrator2/1(Out1) -> Integrator3/1(In1)
  Differentiator2/1(Out1) -> Differentiator3/1(In1)
  Integrator3/1(Out1) -> Down Sample/1
  Differentiator3/1(Out1) -> Out1/1

== system CryoDet6/DspCore/Analysis/FB TriTone 0/TriTone Downconvert/DigitalLO ==
  note: Freq is central frequency in 2^16/pi radians per Tclk
      | but the block downconverter has
      |  shifted the input frequency by Fclk/2
      | and reduced the sample rate by 2
      | so we translate the desired frequency by subtracting 92.5 MHz
  Freq : Inport
  AddSub1 : xbsIndex_r4/AddSub  mode=Subtraction  use_carryin=off  use_carryout=off  en=off  latency=1  precision=User Defined  arith_type="Signed  (2's comp)"  n_bits=16  bin_pt=16  quantization=Truncate  overflow=Wrap  use_behavioral_HDL=off  hw_selection=Fabric  pipelined=off  dbl_ovrd=off  block_type=addsub
  CMult : xbsIndex_r4/CMult  const=2  gui_display_data_type=Fixed-point  const_n_bits=2  const_bin_pt=0  float_type=Single  exp_bits=8  fraction_bits=24  en=off  latency=1  precision=User Defined  arith_type=Unsigned  n_bits=16  bin_pt=16  quantization=Truncate  overflow=Wrap  use_behavioral_HDL=off  mem_type=Distributed RAM  pipeline=off  dbl_ovrd=off  block_type=cmult
  Constant1 : xbsIndex_r4/Constant  const=1.0  gui_display_data_type=Boolean  arith_type=Boolean  n_bits=16  bin_pt=14  preci_type=Single  exp_width=8  frac_width=24  explicit_period=off  period=32*Tclk  equ=P=C  opselect=C  inp2=PCIN>>17  opr=+  inp1=P  carry=CIN  dbl_ovrd=off  block_type=constant
  Constant3 : xbsIndex_r4/Constant  const=0.5  gui_display_data_type=Fixed-point  arith_type=Unsigned  n_bits=16  bin_pt=16  preci_type=Single  exp_width=8  frac_width=24  explicit_period=off  period=1  equ=P=C  opselect=C  inp2=PCIN>>17  opr=+  inp1=P  carry=CIN  dbl_ovrd=off  block_type=constant
  "DDS Compiler 6.0 " : xbsIndex_r4/DDS Compiler 6.0   partspresent=Phase_Generator_and_SIN_COS_LUT  dds_clock_rate=Fclk/1e6  channels=1  mode_of_operation=Standard  modulus=9  parameter_entry=Hardware_Parameters  spurious_free_dynamic_range=45  frequency_resolution=0.4  noise_shaping=None  phase_width=16  output_width=16  output_selection=Sine_and_Cosine  negative_sine=on  negative_cosine=off  amplitude_mode=Unit_Circle  memory_type=Auto  optimization_goal=Speed  dsp48_use=Maximal  resync=off  latency_configuration=Configurable  latency=15  has_phase_out=on  has_aclken=off  has_aresetn=off  explicit_period=on  period=2*Tclk  data_has_tlast=Not_Required  has_tready=off  s_phase_has_tuser=Not_Required  m_data_has_tuser=Not_Required  m_phase_has_tuser=Not_Required  s_phase_tuser_width=1  output_form=Twos_Complement  s_config_sync_mode=On_Vector  phase_increment=Programmable  output_frequency1=0  output_frequency2=0  output_frequency3=0  output_frequency4=0  output_frequency5=0  output_frequency6=0  output_frequency7=0  output_frequency8=0  output_frequency9=0  output_frequency10=0  output_frequency11=0  output_frequency12=0  output_frequency13=0  output_frequency14=0  output_frequency15=0  output_frequency16=0  pinc1='0'  pinc2='0'  pinc3='0'  pinc4='0'  pinc5='0'  pinc6='0'  pinc7='0'  pinc8='0'  pinc9='0'  pinc10='0'  pinc11='0'  pinc12='0'  pinc13='0'  pinc14='0'  pinc15='0'  pinc16='0'  phase_offset=None  phase_offset_angles1=0  phase_offset_angles2=0  phase_offset_angles3=0  phase_offset_angles4=0  phase_offset_angles5=0  phase_offset_angles6=0  phase_offset_angles7=0  phase_offset_angles8=0  phase_offset_angles9=0  phase_offset_angles10=0  phase_offset_angles11=0  phase_offset_angles12=0  phase_offset_angles13=0  phase_offset_angles14=0  phase_offset_angles15=0  phase_offset_angles16=0  poff1='0'  poff2='0'  poff3='0'  poff4='0'  poff5='0'  poff6='0'  poff7='0'  poff8='0'  poff9='0'  poff10='0'  poff11='0'  poff12='0'  poff13='0'  poff14='0'  poff15='0'  poff16='0'  trim_axipin_name=on  simulation_type=hybrid_sim  simulation_model=sysgen:xddsv6_0_cmodel  data_path_portlist={ 's_axis_config_tdata_poff', 's_axis_config_tdata_chan0_poff', 's_axis_config_tdata_pinc', 's_axis_config_tdata_chan0_pinc', 's_axis_phase_tdata_resync', 's_axis_phase_tdata_chan0_resync', 's_axis_phase_tdata_poff', 's_axis_phase_tdata_chan0_poff', 's_axis_phase_tdata_pinc', 's_axis_phase_tdata_chan0_pinc', 's_axis_phase_tdata_phase_in', 'm_axis_data_tdata_sine', 'm_axis_data_tdata_chan0_sine', 'm_axis_data_tdata_cosine', 'm_axis_data_tdata_chan0_cosine', 'm_axis_phase_tdata_phase_out', 'm_axis_phase_tdata_chan0_phase_out'}  por_mode=false  gui_behaviour=Sysgen  ip_name=DDS Compiler  ip_version=6.0  dsptool_ready=true  wrapper_available=true  port_translation_map={ 'aclken' => 'en', 'aresetn' => 'rst' }  ipcore_usecache=true  ipcore_useipmodelcache=true  ipcore_xco_need_fpga_part=true  ipcore_fpga_part=xlipgetpartsetting(gcb, {'kintex7', 'xc7k325t', '-3', 'fbg676'})  ipcore_verbose=false  block_type=dds_compiler_v6_0
  DLO Scope : Scope  NumInputPorts=3
      settings: YMin=0~-1~-1  YMax=3~1~1
  Down Sample : xbsIndex_r4/Down Sample  sample_ratio=2  sample_phase=First Value of Frame  en=off  rst=off  latency=0  dbl_ovrd=off  block_type=dsamp
  Gateway Out : xbsIndex_r4/Gateway Out  inherit_from_input=off  hdl_port=off  rows=1  columns=1  UseAsDAC=off  DACChannel='1'  interface=None  automatic_assignment=on  address_offset=hex2dec('00')  intf_name=''  intf_description=''  timing_constraint=None  locs_specified=off  LOCs={}  io_standard={}  block_type=gatewayout
  Gateway Out1 : xbsIndex_r4/Gateway Out  inherit_from_input=off  hdl_port=off  rows=1  columns=1  UseAsDAC=off  DACChannel='1'  interface=None  automatic_assignment=on  address_offset=hex2dec('00')  intf_name=''  intf_description=''  timing_constraint=None  locs_specified=off  LOCs={}  io_standard={}  block_type=gatewayout
  Gateway Out2 : xbsIndex_r4/Gateway Out  inherit_from_input=off  hdl_port=off  rows=1  columns=1  UseAsDAC=off  DACChannel='1'  interface=None  automatic_assignment=on  address_offset=hex2dec('00')  intf_name=''  intf_description=''  timing_constraint=None  locs_specified=off  LOCs={}  io_standard={}  block_type=gatewayout
  Terminator : Terminator
  Terminator1 : Terminator
  Sin : Outport
  Cos : Outport  Port=2
  wires:
  Gateway Out2/1 -> DLO Scope/1
  Gateway Out/1 -> DLO Scope/2
  Gateway Out1/1 -> DLO Scope/3
  "DDS Compiler 6.0 "/5 -> Gateway Out2/1
  "DDS Compiler 6.0 "/3 -> Gateway Out/1, Cos/1
  "DDS Compiler 6.0 "/2 -> Gateway Out1/1, Sin/1
  "DDS Compiler 6.0 "/4 -> Terminator/1
  "DDS Compiler 6.0 "/1 -> Terminator1/1
  Freq/1 -> AddSub1/1
  Constant3/1 -> AddSub1/2
  CMult/1 -> Down Sample/1
  AddSub1/1 -> CMult/1
  Constant1/1 -> "DDS Compiler 6.0 "/1
  Down Sample/1 -> "DDS Compiler 6.0 "/2

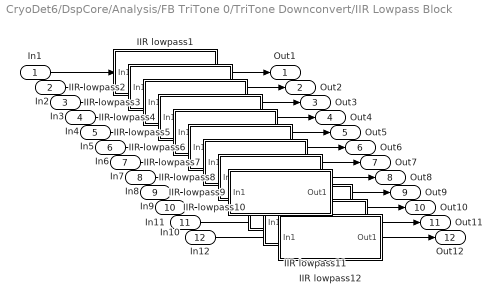
== system CryoDet6/DspCore/Analysis/FB TriTone 0/TriTone Downconvert/IIR Lowpass Block ==
  In1 : Inport
  In2 : Inport  Port=2
  In3 : Inport  Port=3
  In4 : Inport  Port=4
  In5 : Inport  Port=5
  In6 : Inport  Port=6
  In7 : Inport  Port=7
  In8 : Inport  Port=8
  In9 : Inport  Port=9
  In10 : Inport  Port=10
  In11 : Inport  Port=11
  In12 : Inport  Port=12
  IIR lowpass1 : Subsystem
  IIR lowpass10 : Subsystem
  IIR lowpass11 : Subsystem
  IIR lowpass12 : Subsystem
  IIR lowpass2 : Subsystem
  IIR lowpass3 : Subsystem
  IIR lowpass4 : Subsystem
  IIR lowpass5 : Subsystem
  IIR lowpass6 : Subsystem
  IIR lowpass7 : Subsystem
  IIR lowpass8 : Subsystem
  IIR lowpass9 : Subsystem
  Out1 : Outport
  Out2 : Outport  Port=2
  Out3 : Outport  Port=3
  Out4 : Outport  Port=4
  Out5 : Outport  Port=5
  Out6 : Outport  Port=6
  Out7 : Outport  Port=7
  Out8 : Outport  Port=8
  Out9 : Outport  Port=9
  Out10 : Outport  Port=10
  Out11 : Outport  Port=11
  Out12 : Outport  Port=12
  wires:
  In1/1 -> IIR lowpass1/1(In1)
  IIR lowpass1/1(Out1) -> Out1/1
  In2/1 -> IIR lowpass2/1(In1)
  IIR lowpass2/1(Out1) -> Out2/1
  In3/1 -> IIR lowpass3/1(In1)
  IIR lowpass3/1(Out1) -> Out3/1
  In4/1 -> IIR lowpass4/1(In1)
  IIR lowpass4/1(Out1) -> Out4/1
  In5/1 -> IIR lowpass5/1(In1)
  IIR lowpass5/1(Out1) -> Out5/1
  In6/1 -> IIR lowpass6/1(In1)
  IIR lowpass6/1(Out1) -> Out6/1
  In7/1 -> IIR lowpass7/1(In1)
  IIR lowpass7/1(Out1) -> Out7/1
  In8/1 -> IIR lowpass8/1(In1)
  IIR lowpass8/1(Out1) -> Out8/1
  In9/1 -> IIR lowpass9/1(In1)
  IIR lowpass9/1(Out1) -> Out9/1
  In10/1 -> IIR lowpass10/1(In1)
  IIR lowpass10/1(Out1) -> Out10/1
  In11/1 -> IIR lowpass11/1(In1)
  IIR lowpass11/1(Out1) -> Out11/1
  In12/1 -> IIR lowpass12/1(In1)
  IIR lowpass12/1(Out1) -> Out12/1
